simulink model "FFT_Stream_Ex1"  (R2024a)
settings: Solver=VariableStepAuto  StartTime=0.0  StopTime=0.3e-4  RelTol=1e-3
undefined symbols (not defined in the file): None, S, vsva2197, xcvc1902
libraries: aieUtilities x3, aieDSP x1, dspsrcs4 x1, dspxfrm3 x1, vmcUtilities x1
settings Model: Creator=sdegala  LastModifiedBy=abehbood
settings ModelReferenceCC: EnableRefExpFcnMdlSchedulingChecks=on
settings RTWCC: GPUComputeCapability=3.5

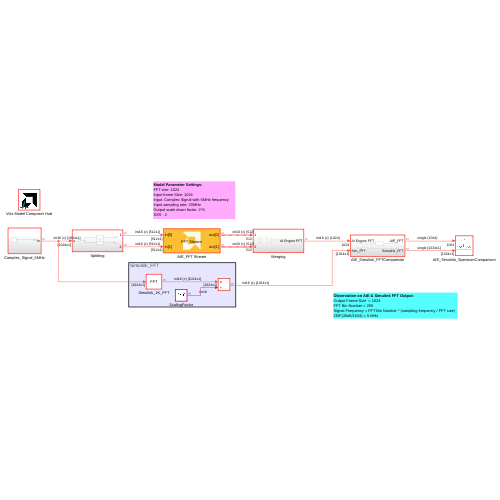
[thumbnail: Simulink's stored preview of the top-level diagram]
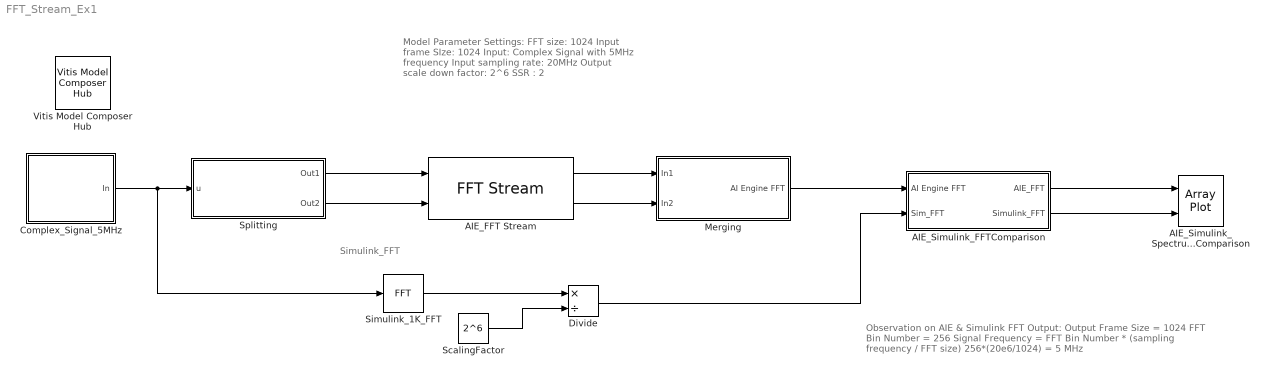
== system FFT_Stream_Ex1 ==
  note: Simulink_FFT
  note: Model Parameter Settings:
      | FFT size: 1024
      | Input frame SIze: 1024
      | Input: Complex Signal with 5MHz frequency
      | Input sampling rate: 20MHz
      | Output scale down factor: 2^6
      | SSR : 2
  note: Observation on AIE & Simulink FFT Output:
      | Output Frame Size = 1024
      | FFT Bin Number = 256
      | Signal Frequency = FFT Bin Number * (sampling frequency / FFT size)
      | 256*(20e6/1024) = 5 MHz
  AIE_FFT Stream : aieDSP/FFT Stream  AIE_VARIANT=1  data_type=cint16  data_out_type=cint16  twiddle_type=cint16  point_size=1024  input_window_size=1024  shift_val=6  rnd_mode=Round symmetrical to infinity  sat_mode=0-None  ssr=2  twiddle_mode=0  use_ssr_widget_kernels=off  casc_length=1  blockJsonConstraints=[]  blockJsonConstraintsInternal=[]  spec=vmc_stream_fft.json  SerializedMaskParamNames=[]  SerializedMaskParamValues=[]  SerializedMaskParamVisibilities=[]  block_type=FFT Stream  SerializedMaskParamDataypes=uint|typename|typename|typename|uint|uint|uint|uint|uint|uint|uint|bool|uint  SerializedMaskParamEnumStrArr=0|0|0|0|0|0|0|Round to positive infinity,Round to negative infinity,Round symmetrical to infinity,Round symmetrical to zero,Round convergent to even,Round convergent to odd|0-None,1-Asymmetric,3-Symmetric|0|0|0|0  SerializedMaskParamEnumValArr=0|0|0|0|0|0|0|2,3,4,5,6,7|0,1,3|0|0|0|0  SerializedMaskParamVectorArr=0|0|0|0|0|0|0|0|0|0|0|0|0
  AIE_Simulink_FFTComparison : Subsystem
  AIE_Simulink_SpectrumComparison : ArrayPlot  NumInputPorts=2  WindowPosition=[915.000000,232.000000,1280.000000,655.000000,]  ScopeFrameLocation=window  CustomXData=[100,1000]  PlotType=Line  AxesScaling=Manual  YLimits=[-22.841163310961967 47.15883668903803]  ShowLegend=on
  Complex_Signal_5MHz : Subsystem
  Divide : Product  Inputs=*/  OutDataTypeStr=int16
  Merging : Subsystem
  ScalingFactor : Constant  Value=2^6  OutDataTypeStr=int16
  Simulink_1K_FFT : dspxfrm3/FFT  FFTImplementation=Auto  CompMethod=Table lookup  TableOpt=NEW  TableOptActive=Speed  BitRevOrder=off  Normalize=off  InheritFFTLength=off  FFTLength=1024  WrapInput=off  roundingMode=Floor  overflowMode=off  firstCoeffDataTypeStr=Inherit: Same word length as input  firstCoeffLastDataTypeStr=Inherit: Same word length as input  prodOutputMode=Binary point scaling  prodOutputWordLength=32  prodOutputFracLength=0  prodOutputDataTypeStr=fixdt(1,32,0)  prodOutputLastDataTypeStr=fixdt(1,32,0)  outputMode=Binary point scaling  outputWordLength=16  outputFracLength=0  outputDataTypeStr=fixdt(1,16,0)  outputMin=[]  outputMax=[]  outputLastDataTypeStr=fixdt(1,16,0)
  Splitting : Subsystem
  Vitis Model Composer Hub : vmcUtilities/Vitis Model Composer Hub  Tag=genX  CodeGeneration=off  StartColumn=1  NumberOfColumns=1  TargetDirectory=./code  exportDesign=off  analyzeDesign=off  validateDesignOnHw=off  ExportType=AI Engines  IpVendor=xilinx.com  IpLibrary=hls  IpVersion=1.0  IpHWLanguage=Verilog  AieCompilerOptions={}  AieSimulatorOptions={}  CreateTestbench=off  TestbenchStackSize=10  RunRtlSim=off  RunCSim=off  RunAieSim=off  AieSimTimeout=50000  RunAieSimProfiling=off  LaunchVitisAnalyzer=off  PlotOutput=off  RunX86Sim=off  X86SimTimeout=10  GenHwImage=off  GenLibadfXo=off  GenHwValidationCode=off  PlatformType=Not Specified  HwSystemType=Baremetal  HwValidationTarget=hw  ProjDevice=xcvc1902-vsva2197-1LP-e-S  ProjDevicePart=xcvc1902-vsva2197-1LP-e-S  AIEType=AIE  SamplePeriod=-1  ClockFrequency=200  DataPathParallelism=1  xilinxfamily=versalaicore  part=xcvc1902  speed=-1LP-e-S  package=vsva2197  directory=./netlist  testbench=off  incr_netlist=off  synthesis_tool=Vivado  clock_wrapper=Clock Enables  dbl_ovrd=According to Block Masks  dcm_input_clock_period=10  sysclk_period=10  simulink_period=1  eval_field=0  LogFileName=''  NThreads=4
  wires:
  Splitting/1(Out1) -> AIE_FFT Stream/1
  Splitting/2(Out2) -> AIE_FFT Stream/2
  AIE_FFT Stream/1 -> Merging/1(In1)
  AIE_FFT Stream/2 -> Merging/2(In2)
  Merging/1(AI Engine FFT) -> AIE_Simulink_FFTComparison/1(AI Engine FFT)
  AIE_Simulink_FFTComparison/1(AIE_FFT) -> AIE_Simulink_SpectrumComparison/1
  AIE_Simulink_FFTComparison/2(Simulink_FFT) -> AIE_Simulink_SpectrumComparison/2
  Divide/1 -> AIE_Simulink_FFTComparison/2(Sim_FFT)
  Complex_Signal_5MHz/1(In) -> Simulink_1K_FFT/1, Splitting/1(u)
  ScalingFactor/1 -> Divide/2
  Simulink_1K_FFT/1 -> Divide/1

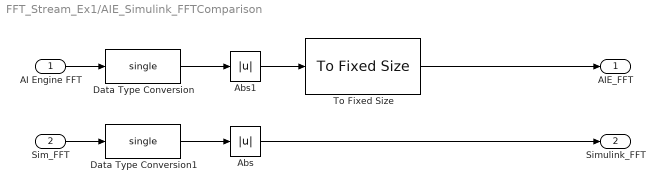
== system FFT_Stream_Ex1/AIE_Simulink_FFTComparison ==
  AI Engine FFT : Inport
  Sim_FFT : Inport  Port=2
  Abs : Abs  SaturateOnIntegerOverflow=off
  Abs1 : Abs  OutDataTypeStr=single  SaturateOnIntegerOverflow=off
  Data Type Conversion : DataTypeConversion  OutDataTypeStr=single  SaturateOnIntegerOverflow=off  RndMeth=Floor
  Data Type Conversion1 : DataTypeConversion  OutDataTypeStr=single  SaturateOnIntegerOverflow=off  RndMeth=Floor
  To Fixed Size : aieUtilities/To Fixed Size  Mode=Stop simulation when input variable-size signal is not full  OutputSize=Inherit: Same as input  CopyMethod=Buffer samples to form output  HasStatusOutput=on
  AIE_FFT : Outport
  Simulink_FFT : Outport  Port=2
  wires:
  AI Engine FFT/1 -> Data Type Conversion/1
  Abs1/1 -> To Fixed Size/1
  To Fixed Size/1 -> AIE_FFT/1
  Abs/1 -> Simulink_FFT/1
  Data Type Conversion/1 -> Abs1/1
  Data Type Conversion1/1 -> Abs/1
  Sim_FFT/1 -> Data Type Conversion1/1

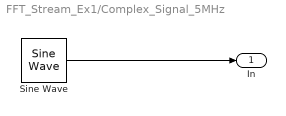
== system FFT_Stream_Ex1/Complex_Signal_5MHz ==
  Sine Wave : dspsrcs4/Sine Wave  Amplitude=1  Frequency=5e6  Phase=0  SampleMode=Discrete  OutComplex=Complex  CompMethod=Table lookup  TableSize=Speed  SampleTime=1/20e6  SamplesPerFrame=1024  ResetState=Restart at time zero  OutputFrames=off  dataType=Fixed-point  wordLen=16  udDataType=sfix(16)  fracBitsMode=User-defined  numFracBits=0  OutDataTypeStr=fixdt(1,16,0)  LastOutDataTypeStr=fixdt(1,16,0)
  In : Outport
  wires:
  Sine Wave/1 -> In/1

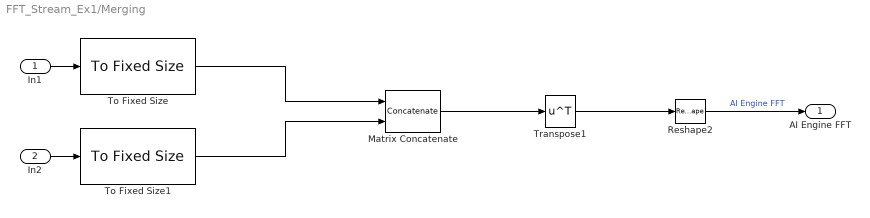
== system FFT_Stream_Ex1/Merging ==
  In1 : Inport
  In2 : Inport  Port=2
  Matrix Concatenate : Concatenate  Mode=Multidimensional array  ConcatenateDimension=2
  Reshape2 : Reshape  OutputDimensions=[1, 10]
  To Fixed Size : aieUtilities/To Fixed Size  Mode=Stop simulation when input variable-size signal is not full  OutputSize=Inherit: Same as input  CopyMethod=Buffer samples to form output  HasStatusOutput=on
  To Fixed Size1 : aieUtilities/To Fixed Size  Mode=Stop simulation when input variable-size signal is not full  OutputSize=Inherit: Same as input  CopyMethod=Buffer samples to form output  HasStatusOutput=on
  Transpose1 : Math  Operator=transpose
  AI Engine FFT : Outport
  wires:
  To Fixed Size1/1 -> Matrix Concatenate/2
  In2/1 -> To Fixed Size1/1
  To Fixed Size/1 -> Matrix Concatenate/1
  Reshape2/1 -> AI Engine FFT/1  "AI Engine FFT"
  In1/1 -> To Fixed Size/1
  Matrix Concatenate/1 -> Transpose1/1
  Transpose1/1 -> Reshape2/1

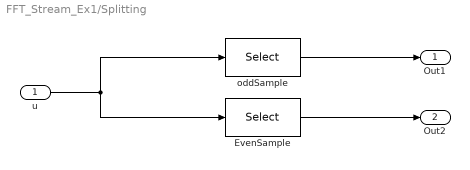
== system FFT_Stream_Ex1/Splitting ==
  u : Inport
  EvenSample : Selector  InputPortWidth=1024  IndexOptions=Index vector (dialog)  Indices=2:2:1024  OutputSizes=1
  oddSample : Selector  InputPortWidth=1024  IndexOptions=Index vector (dialog)  Indices=1:2:1024  OutputSizes=1
  Out1 : Outport
  Out2 : Outport  Port=2
  wires:
  u/1 -> oddSample/1, EvenSample/1
  EvenSample/1 -> Out2/1
  oddSample/1 -> Out1/1
